simulink model "LKAS_DFL"  (R2018b)
settings: Solver=FixedStepDiscrete  StartTime=0.0  StopTime=10.0  FixedStep=0.01  RelTol=1e-3
InitFcn:
  | tmpVer = ver('MATLAB');
  | tmpVer = str2num(tmpVer.Version);
  | % -------------------------------------------------------------------
  | %  MATLAB file generated by Simulink.saveVars on 21-Nov-2019 10:06:14
  | %  MATLAB version: 7.13.0.564 (R2011b)
  | % -------------------------------------------------------------------
  | 
  | 
  | SInt16 = Simulink.AliasType;
  | SInt16.Description = 'Num';
  | if (tmpVer > 7.11)
  | 	SInt16.DataScope = 'Auto';
  | end
  | SInt16.HeaderFile = 'Rte_Type.h';
  | SInt16.BaseType = 'int16';
  | 
  | SInt32 = Simulink.AliasType;
  | SInt32.Description = 'Num';
  | if (tmpVer > 7.11)
  | 	SInt32.DataScope = 'Auto';
  | end
  | SInt32.HeaderFile = 'Rte_Type.h';
  | SInt32.BaseType = 'int32';
  | 
  | SInt8 = Simulink.AliasType;
  | SInt8.Description = 'Num';
  | if (tmpVer > 7.11)
  | 	SInt8.DataScope = 'Auto';
  | end
  | SInt8.HeaderFile = 'Rte_Type.h';
  | SInt8.BaseType = 'int8';
  | 
  | T_A_m2_1024_1_u32 = Simulink.NumericType;
  | T_A_m2_1024_1_u32.Description = 'm2 (square meters  (m2))';
  | if (tmpVer > 7.11)
  | 	T_A_m2_1024_1_u32.DataScope = 'Auto';
  | end
  | T_A_m2_1024_1_u32.HeaderFile = 'Rte_Type.h';
  | T_A_m2_1024_1_u32.DataTypeMode = 'Fixed-point: slope and bias scaling';
  | T_A_m2_1024_1_u32.SignednessBool = false;
  | T_A_m2_1024_1_u32.WordLength = 32;
  | T_A_m2_1024_1_u32.FixedExponent = -10;
  | T_A_m2_1024_1_u32.SlopeAdjustmentFactor = 1;
  | T_A_m2_1024_1_u32.Bias = 0;
  | T_A_m2_1024_1_u32.DataTypeOverride = 'Inherit';
  | T_A_m2_1024_1_u32.IsAlias = true;
  | 
  | T_A_m2_65536_1_u16 = Simulink.NumericType;
  | T_A_m2_65536_1_u16.Description = 'm2 (square meters  (m2))';
  | if (tmpVer > 7.11)
  | 	T_A_m2_65536_1_u16.DataScope = 'Auto';
  | end
  | T_A_m2_65536_1_u16.HeaderFile = 'Rte_Type.h';
  | T_A_m2_65536_1_u16.DataTypeMode = 'Fixed-point: slope and bias scaling';
  | T_A_m2_65536_1_u16.SignednessBool = false;
  | T_A_m2_65536_1_u16.WordLength = 16;
  | T_A_m2_65536_1_u16.FixedExponent = -16;
  | T_A_m2_65536_1_u16.SlopeAdjustmentFactor = 1;
  | T_A_m2_65536_1_u16.Bias = 0;
  | T_A_m2_65536_1_u16.DataTypeOverride = 'Inherit';
  | ... (+4598 lines)
StopFcn:
  | clear  T_A_m2_1024_1_u32 T_A_m2_65536_1_u16 T_A_m2_Float32 T_A_mm2_10_1_u16 T_A_mm2_4_1_s16 T_A_mm2_Float32 T_Cnt_Num_10_1_u32 T_Cnt_Num_1_1_s16 T_Cnt_Num_1_1_s32 T_Cnt_Num_1_1_s8 T_Cnt_Num_1_1_u16 T_Cnt_Num_1_1_u32 T_Cnt_Num_1_1_u8 T_E_J_1_1_s32 T_E_J_Float32 T_E_kJ_128_1_s32 T_E_kJ_Float32 T_E_kwh_10_1_u16 T_E_kwh_Float32 T_Epl_kwhpkm_100_1_u16 T_Epl_kwhpkm_Float32 T_F_N_1_1_s16 T_F_N_Float32 T_I_A_1000_1_u16 T_I_A_1048576_1_s32 T_I_A_2048_1_s16 T_I_A_32_1_s16 T_I_A_Float32 T_I_mA_1_1_s16 T_I_mA_32768_128_s16 T_I_mA_Float32 T_J_kgpm2_128_1_u16 T_J_kgpm2_Float32 T_K_NA_1000_1_s16 T_K_NA_100_1_s16 T_K_NA_100_1_u16 T_K_NA_1024_1_s16 T_K_NA_1024_1_u16 T_K_NA_128_1_s16 T_K_NA_128_1_u16 T_K_NA_128_1_u8 T_K_NA_16777216_1_u32 T_K_NA_16_1_s16 T_K_NA_16_1_u16 T_K_NA_16_1_u8 T_K_NA_1_16_u16 T_K_NA_1_1_s16 T_K_NA_1_1_u16 T_K_NA_1_1_u8 T_K_NA_32768_1_s16 T_K_NA_32768_1_u16 T_K_NA_32_1_s8 T_K_NA_4096_1_u16 T_K_NA_4194304_1_s32 T_K_NA_4194304_1_u16 T_K_NA_65536_1_s32 T_K_NA_65536_1_u16 T_K_NA_8192_1_s16 T_K_NA_8_1_s16 T_K_NA_Float32 T_M_Nm_16_1_s16 T_M_Nm_1_1_s16 T_M_Nm_32768_1_s16 T_M_Nm_32_1_s16 T_M_Nm_4_1_s16 T_M_Nm_512_1_s16 T_M_Nm_Float32 T_P_W_1_4_s16 T_P_W_1_8_s16 T_P_W_Float32 T_P_kW_128_1_s16 T_P_kW_1_8_s16 T_P_kW_8_1_s32 T_P_kW_Float32 T_Pct_pct_1024_1_s32 T_Pct_pct_1024_1_u32 T_Pct_pct_10_1_s16 T_Pct_pct_10_1_u32 T_Pct_pct_128_100_s8 T_Pct_pct_1_1_s16 T_Pct_pct_1_4_u8 T_Pct_pct_255_100_u16 T_Pct_pct_255_100_u8 T_Pct_pct_256_1_s16 T_Pct_pct_256_1_u16 T_Pct_pct_65535_100_u16 T_Pct_pct_Float32 T_R_ohm_1024_1_s16 T_R_ohm_32_1_s16 T_R_ohm_Float32 T_TK_K_16_1_s16 T_TK_K_Float32 T_T_degC_10_400_1_u16 T_T_degC_16_1_s16 T_T_degC_1_40_1_u8 T_T_degC_2_80_1_u8 T_T_degC_Float32 T_U_V_1000_1_u16 T_U_V_10_1_u8 T_U_V_200_1_u8 T_U_V_32_1_s16 T_U_V_4096_1_s16 T_U_V_512_1_s16 T_U_V_65535_8_u16 T_U_V_8192_1_u16 T_U_V_Float32 T_U_mV_1_1_s16 T_U_mV_256_20_u16 T_U_mV_Float32 T_V_l_256_1_s16 T_V_l_4096_1_s16 T_V_l_64_1_s16 T_V_l_65535_100_u16 T_V_l_Float32 T_V_ml_128_1_s16 T_V_ml_1_1_s16 T_V_ml_32768_1_s16 T_V_ml_Float32 T_V_ul_32_1_u16 T_V_ul_Float32 T_Vpl_clpkm_512_1_u16 T_Vpl_clpkm_Float32 T_a_kphps_16_1_s16 T_a_kphps_Float32 T_a_mps2_128_1_s16 T_a_mps2_Float32 T_c_MJpkg_256_1_s16 T_c_MJpkg_Float32 T_c_kJpgpK_1024_1_s16 T_c_kJpgpK_Float32 T_c_kJpkgpK_128_1_u16 T_c_kJpkgpK_Float32 T_chrg_Ah_1_1_s16 T_chrg_Ah_1_1_u16 T_chrg_Ah_1_1_u8 T_chrg_Ah_256_1_u16 T_chrg_Ah_4194304_1_s32 T_chrg_Ah_512_1_u16 T_chrg_Ah_8_1_u16 T_chrg_Ah_Float32 T_cmp_NA_100_1_s16 T_cmp_NA_128_1_s16 T_cmp_NA_16_1_s16 T_cmp_NA_32768_1_u16 T_cmp_NA_Float32 T_d2n_rpmps2_4_1_s16 T_d2n_rpmps2_Float32 T_dPct_pctps_16_1_s16 T_dPct_pctps_256_1_s16 T_dPct_pctps_Float32 T_dT_degCps_128_1_s16 T_dT_degCps_Float32 T_dV_lph_1_1_s16 T_dV_lph_Float32 T_dV_lpm_128_1_s16 T_dV_lpm_32_1_s16 T_dV_lpm_Float32 T_dV_lps_1024_1_u16 T_dV_lps_4_1_u16 T_dV_lps_Float32 T_dV_mlps_1024_1_s16 T_dV_mlps_Float32 T_d_BitField16 T_dm_gps_128_1_s16 T_dm_gps_128_1_u16 T_dm_gps_256_1_u16 T_dm_gps_Float32 T_dm_mgps_1_1_s16 T_dm_mgps_Float32 T_dn_rpmps_1_1_s16 T_dn_rpmps_2_1_s16 T_dn_rpmps_Float32 T_dp_Paps_1_1_s16 T_dp_Paps_Float32 T_dp_kPaps_1_1_s16 T_dp_kPaps_8_1_s16 T_dp_kPaps_Float32 T_dphi_degps_128_1_s16 T_dphi_degps_8_1_s16 T_dphi_degps_Float32 T_dr_ps_256_1_s16 T_dr_ps_Float32 T_drho_mgplps_1_2_s16 T_drho_mgplps_Float32 T_e_NA_1_1_u8 T_f_Hz_1_1_u16 T_f_Hz_1_1_u32 T_f_Hz_64_1_u16 T_f_Hz_8_1_s16 T_f_Hz_Float32 T_g_BitField32 T_l_km_16_1_s16 T_l_km_1_1_u16 T_l_km_1_1_u32 T_l_km_Float32 T_l_m_1024_1_s16 T_l_m_16_1_s16 T_l_m_1_1_u32 T_l_m_Float32 T_l_mm_16_1_s16 T_l_mm_1_1_u16 T_l_mm_4096_1_s16 T_l_mm_4_1_u8 T_l_mm_64_1_s16 T_l_mm_Float32 T_m_g_1_1_s16 T_m_g_2048_1_s16 T_m_g_32_1_u16 T_m_g_Float32 T_m_kg_1024_1_s16 T_m_kg_1_1_s16 T_m_kg_1_1_u32 T_m_kg_Float32 T_m_mg_128_1_s16 T_m_mg_32_1_s16 T_m_mg_Float32 T_n_rpm_1_1_s16 T_n_rpm_1_25_u8 T_n_rpm_256_50_u16 T_n_rpm_2_25_u8 T_n_rpm_4_1_u16 T_n_rpm_Float32 T_p_MPa_64_1_s16 T_p_MPa_Float32 T_p_Pa_1_1_s16 T_p_Pa_Float32 T_p_kPa_1_10_u16 T_p_kPa_1_1_s16 T_p_kPa_1_1_u8 T_p_kPa_256_1_u16 T_p_kPa_32_1_u16 T_p_kPa_64_1_s16 T_p_kPa_Float32 T_phi_deg_100_1_s16 T_phi_deg_1024_1_s16 T_phi_deg_128_1_s16 T_phi_deg_1_1_u8 T_phi_deg_256_1_s16 T_phi_deg_2_1_s8 T_phi_deg_32_1_s16 T_phi_deg_512_6_s32 T_phi_deg_Float32 T_phi_rad_2048_1_s16 T_phi_rad_Float32 T_r_NA_1024_1_s16 T_r_NA_1024_1_u16 T_r_NA_16384_1_s16 T_r_NA_16_1_s16 T_r_NA_256_1_s8 T_r_NA_256_1_u16 T_r_NA_32768_1_u16 T_r_NA_32_1_u16 T_r_NA_4096_1_s16 T_r_NA_65535_2_u16 T_r_NA_8192_1_u16 T_r_NA_Float32 T_rho_gpl_8192_1_s16 T_rho_gpl_Float32 T_rho_kgpm3_16_1_s16 T_rho_kgpm3_Float32 T_rho_mgpl_1_1_s16 T_rho_mgpl_64_1_s16 T_rho_mgpl_Float32 T_t_hour_1_1_s16 T_t_hour_Float32 T_t_m_1_1_u16 T_t_m_Float32 T_t_ms_1_1_s16 T_t_ms_1_1_u16 T_t_ms_1_1_u32 T_t_ms_4096_1_s16 T_t_ms_64_1_s16 T_t_ms_Float32 T_t_s_1000_1_s16 T_t_s_100_1_s16 T_t_s_10_1_s16 T_t_s_10_1_u16 T_t_s_1_1_s16 T_t_s_1_1_u16 T_t_s_1_1_u32 T_t_s_Float32 T_t_us_10_1_u32 T_t_us_1_1_s16 T_t_us_1_1_u32 T_t_us_1_4_u16 T_t_us_Float32 T_v_kph_1_1_u8 T_v_kph_64_1_s16 T_v_kph_64_1_u16 T_v_kph_Float32 T_v_mps_256_1_s16 T_v_mps_Float32 T_w_radps_32_1_s16 T_w_radps_Float32 T_y_BitField8 T_y_BitFieldDiagProgress T_y_BitFieldDiagStatus T_y_NA_1_1_u8 SInt16 SInt32 SInt8 T_BOOLEAN UInt16 UInt32 UInt8 s16 s32 s8 u16 u32 u8
model workspace (MAT data in the model file):
  MCOS : class17 (value not decoded)
  MCOS : class17 (value not decoded)
  MCOS : class17 (value not decoded)
  MCOS : class17 (value not decoded)
  MCOS : class17 (value not decoded)
  MCOS : class17 (value not decoded)
  MCOS : class17 (value not decoded)
  MCOS : class17 (value not decoded)
  MCOS : class17 (value not decoded)
  MCOS : class17 (value not decoded)
  MCOS : class17 (value not decoded)
  MCOS : class17 (value not decoded)
  MCOS : class17 (value not decoded)
  MCOS : class17 (value not decoded)
  MCOS : class17 (value not decoded)
  MCOS : class17 (value not decoded)
  MCOS : class17 (value not decoded)
  MCOS : class17 (value not decoded)
  MCOS : class17 (value not decoded)
  MCOS : class17 (value not decoded)
  MCOS : class17 (value not decoded)
  MCOS : class17 (value not decoded)
  MCOS : class17 (value not decoded)
  MCOS : class17 (value not decoded)
  MCOS : class17 (value not decoded)
  MCOS : class17 (value not decoded)
  MCOS : class17 (value not decoded)
  MCOS : class17 (value not decoded)
  MCOS : class17 (value not decoded)
  MCOS : class17 (value not decoded)
  MCOS : class17 (value not decoded)
  MCOS : class17 (value not decoded)
  MCOS : class17 (value not decoded)
  MCOS : class17 (value not decoded)
  MCOS : class17 (value not decoded)
  MCOS : class17 (value not decoded)
  MCOS : class17 (value not decoded)
  MCOS : class17 (value not decoded)
  MCOS : class17 (value not decoded)
  MCOS : class17 (value not decoded)
  MCOS : class17 (value not decoded)
  MCOS : class17 (value not decoded)
  MCOS : class17 (value not decoded)
  MCOS : class17 (value not decoded)
  MCOS : class17 (value not decoded)
  MCOS : class17 (value not decoded)
  MCOS : class17 (value not decoded)
  MCOS : class17 (value not decoded)
  MCOS : class17 (value not decoded)
  MCOS : class17 (value not decoded)
  MCOS : class17 (value not decoded)
  MCOS : class17 (value not decoded)
  MCOS : class17 (value not decoded)
  MCOS : class17 (value not decoded)
  MCOS : class17 (value not decoded)
  MCOS : class17 (value not decoded)
  MCOS : class17 (value not decoded)
  MCOS : class17 (value not decoded)
  MCOS : class17 (value not decoded)
  MCOS : class17 (value not decoded)
  MCOS : class17 (value not decoded)
  MCOS : class17 (value not decoded)
  MCOS : class17 (value not decoded)
  MCOS : class17 (value not decoded)
  MCOS : class17 (value not decoded)
  MCOS : class17 (value not decoded)
  MCOS : class17 (value not decoded)
  MCOS : class17 (value not decoded)
  MCOS : class17 (value not decoded)
  MCOS : class17 (value not decoded)
  MCOS : class17 (value not decoded)
  MCOS : class17 (value not decoded)
  MCOS : class17 (value not decoded)
  MCOS : class17 (value not decoded)
  MCOS : class17 (value not decoded)
  MCOS : class17 (value not decoded)
  MCOS : class17 (value not decoded)
  MCOS : class17 (value not decoded)
  MCOS : class17 (value not decoded)
  MCOS : class17 (value not decoded)
  MCOS : class17 (value not decoded)
  MCOS : class17 (value not decoded)
  MCOS : class17 (value not decoded)
  MCOS : class17 (value not decoded)
  MCOS : class17 (value not decoded)
  MCOS : class17 (value not decoded)
  MCOS : class17 (value not decoded)
  MCOS : class17 (value not decoded)
  MCOS : class17 (value not decoded)
  MCOS : class17 (value not decoded)
  MCOS : class17 (value not decoded)
  MCOS : class17 (value not decoded)
  MCOS : class17 (value not decoded)
  MCOS : class17 (value not decoded)
  MCOS : class17 (value not decoded)
  MCOS : class17 (value not decoded)
  MCOS : class17 (value not decoded)
  MCOS : class17 (value not decoded)
  MCOS : class17 (value not decoded)
  MCOS : class17 (value not decoded)
  MCOS : class17 (value not decoded)
  MCOS : class17 (value not decoded)
  MCOS : class17 (value not decoded)
  MCOS : class17 (value not decoded)
  MCOS : class17 (value not decoded)
  MCOS : class17 (value not decoded)
undefined symbols (not defined in the file): LKA_CarWidth, LKA_SampleTime, LKA_StrRatio_C, LKA_Veh2CamL_C, LKA_Veh2CamW_C, LKA_WhlBaseL_C, LL_CompSWA_C, LL_CrvtPrvwT_C, LL_DesDvt_C, LL_DvtComp_C, LL_DvtPrvwT_C, LL_DvtSpdDet_vDvtSpdMin_C, LL_HdAgExT_C, LL_HdAgPrvwT_C, LL_LAccMax_C, LL_LAccRMax_C, LL_Laneline_Select, LL_LDW_EarliestWarnLine_C, LL_LDW_LatestWarnLine_C, LL_LDWS_SUPPRESS_HEADING, LL_LFClb_TFC_DiffCtlBalance, LL_LFClb_TFC_DiffCtrlMaxSWA, LL_LFClb_TFC_DiffCtrlRatio, LL_LFClb_TFC_facmGainLutGain1_C, LL_LFClb_TFC_facmGainLutGain2_C, LL_LFClb_TFC_facmIntegRatio, LL_LFClb_TFC_facmKlat_C, LL_LFClb_TFC_FfCtlRatio_C, LL_LFClb_TFC_phiIntegCtlMaxSWA_C, LL_LFClb_TFC_tiKlatPrvwT_C, LL_LFClb_TFC_vGainLutVehSpdLwr_C, LL_LFClb_TFC_vGainLutVehSpdUpr_C, LL_LKA_EarliestWarnLine_C, LL_LKA_LatestWarnLine_C, LL_LKA_SWATrq_Kf_Switch, LL_LKA_SWATrq_KfA, LL_LKA_SWATrq_KfB, LL_LKA_SWATrq_KiA, LL_LKA_SWATrq_KiB, LL_LKA_SWATrq_KiMax, LL_LKA_SWATrq_Kp, LL_LKAExPrcs_ExitC0Dvt, LL_LKAExPrcs_ExitC0Swt, LL_LKAExPrcs_tiExitTime1, LL_LKAExPrcs_tiExitTime2, LL_LKAExPrcs_tiExitTime3, LL_LKAS_OUT_OF_CONTROL_LAT_VEL, LL_LKAS_OUT_OF_CONTROL_TTLC, LL_LKASWASyn_M0, LL_LKASWASyn_M1, LL_LKASWASyn_M2, LL_LKASWASyn_M3K, LL_LKASWASyn_SWAaddMax, LL_LKASWASyn_T2, LL_LKASWASyn_tiTrqSwaRtTime, LL_LKASWASyn_tiTrqSwaTime, LL_LKASWASyn_TrqMax, LL_LKASWASyn_TrqSwaAddSwt, LL_LKASWASyn_TrqSwaRateDiff, LL_LSpdCompT_C ... (+42)
libraries: simulink x137, dspstat3 x3, simulink_extras x1
(part 9 of 19)

== system LKAS_DFL/LKAS/LL/LLOn/LKA/Driver Torque Addition (DTA)/Subsystem ==
  DTA_bsInInfoSyn : Inport
  DTA_bsLFClb : Inport  Port=2
  Enable : EnablePort
      settings: AttributesFormatString=states = %<StatesWhenEnabling>
  Add : Sum
  Bus Selector2 : BusSelector  OutputSignals=bsVehMovInfo.ESC_VehSpd,bsEPSInfo.EPS_SW_Trq,bsLaneInfo.bsL0Info.L0_C0,bsLaneInfo.bsR0Info.R0_C0
  Bus Selector4 : BusSelector  OutputSignals=bsLKAClb.LL_LKASWAClb.LL_LKASWASyn_SWAaddMax,bsLKAClb.LL_LKASWAClb.LL_LKASWASyn_TrqMax,bsLKAClb.LL_LKASWAClb.LL_LKASWASyn_TrqSwaAddSwt,bsLKAClb.LL_LKASWAClb.LL_LKASWASyn_tiTrqSwaTime,bsLKAClb.LL_LKASWAClb.LL_LKASWASyn_tiTrqSwaRtTime,bsLKAClb.LL_LKASWAClb.LL_LKASWASyn_TrqSwaRateDiff,bsConstantClb.LKA_SampleTime
  Constant1 : Constant  Value=5  OutDataTypeStr=single
  Constant2 : Constant  Value=-5  OutDataTypeStr=single
  Divide1 : Product  Inputs=***
  Divide3 : Product  Inputs=**
  DriverSwaTrqAdd : MATLAB Function  TreatAsAtomicUnit=on
  LowPass : Subsystem
  LowPass1 : Subsystem
  Rate Limiter Dynamic : simulink/Discontinuities/Rate Limiter Dynamic
      settings: SourceProductName=Simulink
  Saturation : Saturate  UpperLimit=30  LowerLimit=-30
      settings: AttributesFormatString="Min = %<LowerLimit>  Max = %<UpperLimit>"
  Out1 : Outport  OutputWhenDisabled=reset  InitialOutput=0
      settings: AttributesFormatString=%<OutputWhenDisabled> = %<InitialOutput>
  wires:
  Add/1 -> Rate Limiter Dynamic/2
  Bus Selector4/3 -> Divide3/1, Divide1/1  "<LL_LKASWASyn_TrqSwaAddSwt>"
  LowPass1/1(y) -> Saturation/1  "SWARateAdd"
  Divide3/1 -> Add/1  "TrqSWAAdd"
  Constant2/1 -> Rate Limiter Dynamic/3
  Bus Selector4/1 -> DriverSwaTrqAdd/5(swaaddmax)  "<LL_LKASWASyn_SWAaddMax>"
  Constant1/1 -> Rate Limiter Dynamic/1
  DriverSwaTrqAdd/1(Swaadd) -> LowPass/2(u)  "TrqSWAAddRaw"
  Rate Limiter Dynamic/1 -> Out1/1
  Saturation/1 -> Divide1/2
  DTA_bsInInfoSyn/1 -> Bus Selector2/1
  Bus Selector4/4 -> LowPass/1(T)  "<LL_LKASWASyn_tiTrqSwaTime>"
  LowPass/1(y) -> Divide3/2, LowPass1/2(u)  "TrqSWAAdd"
  Divide1/1 -> Add/2  "SWARateAdd"
  Bus Selector2/2 -> DriverSwaTrqAdd/2(trq)  "<EPS_SW_Trq>"
  Bus Selector2/4 -> DriverSwaTrqAdd/4(r0c0)  "<R0_C0>"
  Bus Selector4/6 -> Divide1/3  "<LL_LKASWASyn_TrqSwaRateDiff>"
  Bus Selector2/1 -> DriverSwaTrqAdd/1(spd)  "<ESC_VehSpd>"
  Bus Selector4/5 -> LowPass1/1(T)  "<LL_LKASWASyn_tiTrqSwaRtTime>"
  Bus Selector2/3 -> DriverSwaTrqAdd/3(l0c0)  "<L0_C0>"
  Bus Selector4/7 -> LowPass1/3(dT), LowPass/3(dT)  "<LKA_SampleTime>"
  Bus Selector4/2 -> DriverSwaTrqAdd/6(trqmax)  "<LL_LKASWASyn_TrqMax>"
  DTA_bsLFClb/1 -> Bus Selector4/1

== system LKAS_DFL/LKAS/LL/LLOn/LKA/Driver Torque Addition (DTA)/Subsystem1 ==
  DTA_bsInInfoSyn : Inport
  DTA_bsLFClb : Inport  Port=2
  Add1 : Sum  Inputs=-+
  Bus Selector : BusSelector  OutputSignals=bsEPSInfo.EPS_SW_Trq
  Bus Selector1 : BusSelector  OutputSignals=bsLKAClb.LL_LKASWAClb.LL_LKASWASyn_M3K,bsLKAClb.LL_LKASWAClb.LL_LKASWASyn_M0,bsLKAClb.LL_LKASWAClb.LL_LKASWASyn_M1,bsLKAClb.LL_LKASWAClb.LL_LKASWASyn_M2,bsLKAClb.LL_LKASWAClb.LL_LKASWASyn_T2
  Divide : Product  Inputs=**
  MATLAB Function : MATLAB Function  TreatAsAtomicUnit=on
  Moving Standard Deviation2 : Subsystem  TreatAsAtomicUnit=on
      mask Display: disp(['Moving' char(10) 'Standard' char(10) 'Deviation']);
  Saturation1 : Saturate  UpperLimit=0.2  LowerLimit=0
      settings: AttributesFormatString="Min = %<LowerLimit>  Max = %<UpperLimit>"
  Saturation2 : Saturate  UpperLimit=1  LowerLimit=0
      settings: AttributesFormatString="Min = %<LowerLimit>  Max = %<UpperLimit>"
  TickTime (TTime) : Subsystem
      mask Display:
      | port_label('output', 1, 'TTime');
      | color('blue');
      | text(0.98,0.9,'VCDC Block','horizontalAlignment','right');
      | color('black');
      | text(0.5,0.55,'Tick Time','horizontalAlignment','center');
      | text(0.5,0.4,'(TTime)','horizontalAlignment','center');
  Out1 : Outport
  wires:
  Bus Selector1/2 -> MATLAB Function/1(M0)  "<LL_LKASWASyn_M0>"
  Bus Selector1/3 -> MATLAB Function/2(M1)  "<LL_LKASWASyn_M1>"
  [PT1] -> MATLAB Function/4(T1)
  [T] -> MATLAB Function/6(T)
  Saturation1/1 -> Add1/1  "M3"
  MATLAB Function/1(M) -> Add1/2
  Bus Selector1/5 -> MATLAB Function/5(T2)  "<LL_LKASWASyn_T2>"
  TickTime (TTime)/1(Out1) -> [T]
  Divide/1 -> Saturation1/1
  Add1/1 -> Saturation2/1
  Bus Selector1/1 -> Divide/2  "<LL_LKASWASyn_M3K>"
  Bus Selector1/4 -> MATLAB Function/3(M2)  "<LL_LKASWASyn_M2>"
  Bus Selector/1 -> Moving Standard Deviation2/1(In1)  "<EPS_SW_Trq>"
  Moving Standard Deviation2/1(Out1) -> Divide/1
  DTA_bsInInfoSyn/1 -> Bus Selector/1
  DTA_bsLFClb/1 -> Bus Selector1/1
  Saturation2/1 -> Out1/1

== system LKAS_DFL/LKAS/LL/LLOn/LKA/LKA Exit Processing (LKAExPrcs)/Exit Time 1 ==
  bsLKAInPInfo : Inport
  bsLKAClb : Inport  Port=2
  Abs : Abs
  Add : Sum
  Add2 : Sum  OutDataTypeStr=single
  Bus Selector1 : BusSelector  OutputSignals=bsConstantClb.LKA_SampleTime,bsLKAClb.LL_LKAExPrcs.LL_LKAExPrcs_tiExitTime1
  Bus Selector2 : BusSelector  OutputSignals=bsPrCrvtInfo.crPrvwCrvt
  Constant : Constant  Value=0.004  OutDataTypeStr=single
  Constant1 : Constant  Value=0.5  OutDataTypeStr=single
  Divide : Product  Inputs=***/
  Memory : Memory  InheritSampleTime=on
  Relational Operator4 : RelationalOperator  OutDataTypeStr=boolean  RndMeth=Nearest
  Saturation : Saturate  UpperLimit=0.004  LowerLimit=0
      settings: AttributesFormatString="Min = %<LowerLimit>  Max = %<UpperLimit>"
  Saturation2 : Saturate  UpperLimit=20  LowerLimit=0
      settings: AttributesFormatString="Min = %<LowerLimit>  Max = %<UpperLimit>"
  Exit1 : Outport
  wires:
  Saturation2/1 -> Relational Operator4/1, Memory/1
  Bus Selector1/1 -> Add2/1  "<LKA_SampleTime>"
  bsLKAClb/1 -> Bus Selector1/1
  Add2/1 -> Saturation2/1
  Memory/1 -> Add2/2
  Relational Operator4/1 -> Exit1/1
  bsLKAInPInfo/1 -> Bus Selector2/1
  Constant/1 -> Divide/4
  Constant1/1 -> Divide/2
  Bus Selector2/1 -> Abs/1  "<crPrvwCrvt>"
  Divide/1 -> Add/2
  Abs/1 -> Saturation/1
  Add/1 -> Relational Operator4/2
  Saturation/1 -> Divide/3
  Bus Selector1/2 -> Add/1, Divide/1  "<LL_LKAExPrcs_tiExitTime1>"

== system LKAS_DFL/LKAS/LL/LLOn/LKA/LKA Exit Processing (LKAExPrcs)/Exit Time 2 ==
  bsLKAClb : Inport
  bsLKAInPInfo : Inport  Port=2
  T1 : Inport  Port=3
  Abs : Abs
  Abs2 : Abs
  Abs3 : Abs
  Add1 : Sum
  Add2 : Sum  OutDataTypeStr=single
  Add3 : Sum  Inputs=+-
  Bus Selector1 : BusSelector  OutputSignals=bsPrCrvtInfo.crPrvwCrvt
  Bus Selector3 : BusSelector  OutputSignals=bsConstantClb.LKA_SampleTime,bsConstantClb.LKA_CarWidth,bsLKAClb.LL_LKAExPrcs.LL_LKAExPrcs_tiExitTime2
  Bus Selector4 : BusSelector  OutputSignals=bsDvtInfo.ILftDvt,bsDvtInfo.IRgtDvt,LaneWidth
  Constant : Constant  Value=0.004  OutDataTypeStr=single
  Constant1 : Constant  Value=0.5  OutDataTypeStr=single
  Divide : Product  Inputs=***/
  Gain : Gain  Gain=1/6
  Logical Operator1 : Logic  Inputs=3  AllPortsSameDT=off  OutDataTypeStr=boolean
  Memory : Memory  InheritSampleTime=on
  Relational Operator2 : RelationalOperator  OutDataTypeStr=boolean  RndMeth=Nearest
  Relational Operator3 : RelationalOperator  OutDataTypeStr=boolean  RndMeth=Nearest
  Relational Operator4 : RelationalOperator  OutDataTypeStr=boolean  RndMeth=Nearest
  Saturation : Saturate  UpperLimit=0.004  LowerLimit=0
      settings: AttributesFormatString="Min = %<LowerLimit>  Max = %<UpperLimit>"
  Saturation2 : Saturate  UpperLimit=12  LowerLimit=0
      settings: AttributesFormatString="Min = %<LowerLimit>  Max = %<UpperLimit>"
  Sum Condition1 : Subsystem
  Exit2 : Outport
  wires:
  Add3/1 -> Gain/1
  Bus Selector4/3 -> Add3/1  "<LaneWidth>"
  Bus Selector4/2 -> Abs3/1  "<IRgtDvt>"
  Bus Selector4/1 -> Abs2/1  "<ILftDvt>"
  Saturation2/1 -> Relational Operator4/1, Memory/1
  Gain/1 -> Relational Operator2/2, Relational Operator3/2
  Abs3/1 -> Relational Operator3/1
  Relational Operator2/1 -> Logical Operator1/2
  Abs2/1 -> Relational Operator2/1
  Relational Operator3/1 -> Logical Operator1/3
  Logical Operator1/1 -> Sum Condition1/Enable
  Add2/1 -> Saturation2/1
  Relational Operator4/1 -> Logical Operator1/1
  Memory/1 -> Add2/2
  Bus Selector3/1 -> Sum Condition1/1(Sample Time), Add2/1  "<LKA_SampleTime>"
  T1/1 -> Relational Operator4/2
  Sum Condition1/1(Out) -> Exit2/1
  bsLKAInPInfo/1 -> Bus Selector1/1, Bus Selector4/1
  Bus Selector1/1 -> Abs/1  "<crPrvwCrvt>"
  Add1/1 -> Sum Condition1/2(Time Exit 2)
  Constant/1 -> Divide/4
  Abs/1 -> Saturation/1
  Constant1/1 -> Divide/2
  Divide/1 -> Add1/2
  Saturation/1 -> Divide/3
  bsLKAClb/1 -> Bus Selector3/1
  Bus Selector3/2 -> Add3/2  "<LKA_CarWidth>"
  Bus Selector3/3 -> Add1/1, Divide/1  "<LL_LKAExPrcs_tiExitTime2>"

== system LKAS_DFL/LKAS/LL/LLOn/LKA/LKA Exit Processing (LKAExPrcs)/Exit Time 3 ==
  bsLKAInPInfo : Inport
  bsLKAClb : Inport  Port=2
  T1 : Inport  Port=3
  Abs4 : Abs
  Add : Sum  Inputs=+-
  Add2 : Sum  OutDataTypeStr=single
  Add6 : Sum
  Bus Selector3 : BusSelector  OutputSignals=bsConstantClb.LKA_SampleTime,bsConstantClb.LKA_CarWidth,bsLKAClb.LL_LKAExPrcs.LL_LKAExPrcs_tiExitTime3,bsLKAClb.LL_LKAExPrcs.LL_LKAExPrcs_ExitC0Dvt,bsLKAClb.LL_LKAExPrcs.LL_LKAExPrcs_ExitC0Swt
  Bus Selector4 : BusSelector  OutputSignals=bsPrCrvtInfo.crPrvwCrvt
  Bus Selector5 : BusSelector  OutputSignals=LaneWidth,bsDvtInfo.ILftDvt,bsDvtInfo.IRgtDvt
  Constant : Constant  Value=0.004  OutDataTypeStr=single
  Constant7 : Constant  Value=2  OutDataTypeStr=single
  Divide1 : Product  Inputs=**/
  Gain : Gain  Gain=1/3
  Logical Operator1 : Logic  Inputs=3  AllPortsSameDT=off  OutDataTypeStr=boolean
  Logical Operator2 : Logic  Inputs=4  AllPortsSameDT=off  OutDataTypeStr=boolean
  Memory : Memory  InheritSampleTime=on
  Moving Standard Deviation1 : Subsystem  TreatAsAtomicUnit=on
      mask Display: disp(['Moving' char(10) 'Standard' char(10) 'Deviation']);
  Moving Standard Deviation2 : Subsystem  TreatAsAtomicUnit=on
      mask Display: disp(['Moving' char(10) 'Standard' char(10) 'Deviation']);
  Relational Operator2 : RelationalOperator  OutDataTypeStr=boolean  RndMeth=Nearest
  Relational Operator3 : RelationalOperator  OutDataTypeStr=boolean  RndMeth=Nearest
  Relational Operator4 : RelationalOperator  OutDataTypeStr=boolean  RndMeth=Nearest
  Relational Operator5 : RelationalOperator  Operator=<=  OutDataTypeStr=boolean  RndMeth=Nearest
  Relational Operator6 : RelationalOperator  Operator=<=  OutDataTypeStr=boolean  RndMeth=Nearest
  Saturation : Saturate  UpperLimit=0.004  LowerLimit=0
      settings: AttributesFormatString="Min = %<LowerLimit>  Max = %<UpperLimit>"
  Saturation2 : Saturate  UpperLimit=10  LowerLimit=0
      settings: AttributesFormatString="Min = %<LowerLimit>  Max = %<UpperLimit>"
  Sum Condition : Subsystem
  Sum Condition1 : Subsystem
  Exit3 : Outport
  wires:
  Gain/1 -> Relational Operator2/2, Relational Operator3/2
  Bus Selector5/1 -> Add/1  "<LaneWidth>"
  Bus Selector5/2 -> Moving Standard Deviation2/1(In1), Relational Operator2/1  "<ILftDvt>"
  Bus Selector5/3 -> Relational Operator3/1, Moving Standard Deviation1/1(In1)  "<IRgtDvt>"
  T1/1 -> Relational Operator4/2
  [LKA_SampleTime] -> Add2/1
  Memory/1 -> Add2/2
  Add2/1 -> Saturation2/1
  Relational Operator4/1 -> Logical Operator1/1
  Saturation2/1 -> Relational Operator4/1, Memory/1
  Logical Operator1/1 -> Logical Operator2/1
  Relational Operator3/1 -> Logical Operator1/3
  Relational Operator2/1 -> Logical Operator1/2
  Add/1 -> Gain/1
  bsLKAClb/1 -> Bus Selector3/1
  Logical Operator2/1 -> Exit3/1
  Moving Standard Deviation2/1(Out1) -> Relational Operator5/1
  Relational Operator5/1 -> Sum Condition/Enable
  Sum Condition/1(Out) -> Logical Operator2/3
  Sum Condition1/1(Out) -> Logical Operator2/2
  Relational Operator6/1 -> Sum Condition1/Enable
  Add6/1 -> Sum Condition/2(In1), Sum Condition1/2(In1)
  Moving Standard Deviation1/1(Out1) -> Relational Operator6/1
  bsLKAInPInfo/1 -> Bus Selector4/1, Bus Selector5/1
  Constant/1 -> Divide1/3
  Divide1/1 -> Add6/2
  Abs4/1 -> Saturation/1
  Saturation/1 -> Divide1/2
  Bus Selector4/1 -> Abs4/1  "<crPrvwCrvt>"
  Constant7/1 -> Divide1/1
  [LKA_SampleTime] -> Sum Condition1/1(In), Sum Condition/1(In)
  Bus Selector3/5 -> Logical Operator2/4  "<LL_LKAExPrcs_ExitC0Swt>"
  Bus Selector3/4 -> Relational Operator6/2, Relational Operator5/2  "<LL_LKAExPrcs_ExitC0Dvt>"
  Bus Selector3/3 -> Add6/1  "<LL_LKAExPrcs_tiExitTime3>"
  Bus Selector3/2 -> Add/2  "<LKA_CarWidth>"
  Bus Selector3/1 -> [LKA_SampleTime]  "<LKA_SampleTime>"

== system LKAS_DFL/LKAS/LL/LLOn/LKA/LKA Motion Planning (LKAMP) /LKA Motion Planning Calculation (LKAMPCal) ==
  LKAMPCal_bsLKAInPInfo : Inport
  LKAMPCal_bsLKAClb : Inport  Port=2
  Action Port : ActionPort  InitializeStates=reset
      settings: AttributesFormatString=states = %<InitializeStates>
  Bus Creator : BusCreator  Inputs=6
  Bus Creator3 : BusCreator  Inputs=5
  Bus Selector : BusSelector  OutputSignals=MPInP_stLDDir,MPInP_tiTTLCIni,MPInP_vVehSpdIni,MPInP_phiSWAIni,MPInP_phiPrvwHdAgIni,MPInP_phiHdAgIni,MPInP_phiHdAgMax,MPInP_lDvtIni,UndrLim_dphiSWARMax,StbFacm_SY
  Bus Selector1 : BusSelector  OutputSignals=bsConstantClb.LKA_WhlBaseL_C,bsConstantClb.LKA_StrRatio_C,bsLKAClb.LL_DesDvt_C,bsLKAClb.LL_lStpLngth_C
  Bus Selector3 : BusSelector  OutputSignals=signal1,signal2,signal3,signal4,signal5
  MATLAB Function : MATLAB Function  TreatAsAtomicUnit=on
  Memory{,1..4} (5 alike) : Memory  InheritSampleTime=on
  Time Division (TDiv) : Subsystem
  Time Division (TDiv)1 : Subsystem
  Time Division (TDiv)2 : Subsystem
  Time Division (TDiv)3 : Subsystem
  Time Division (TDiv)4 : Subsystem
  LKAMPCal_bsLKAMPCalOut : Outport
      settings: AttributesFormatString=%<OutputWhenDisabled> = %<InitialOutput>
  wires:
  Time Division (TDiv)4/1(Out2) -> Bus Creator3/5
  Time Division (TDiv)3/1(Out2) -> Bus Creator3/4
  Time Division (TDiv)2/1(Out2) -> Bus Creator3/3
  Time Division (TDiv)1/1(Out2) -> Bus Creator3/2
  Time Division (TDiv)/1(Out1) -> Bus Creator3/1
  Memory4/1 -> Time Division (TDiv)4/1(TDiv_bsTDivInfoOut1)
  MATLAB Function/11(K1K2Det_bsTDivInfoOut_Ph2SWAIni) -> Memory4/1
  MATLAB Function/10(K1K2Det_bsTDivInfoOut_Ph2DvtEnd) -> Memory3/1
  Memory3/1 -> Time Division (TDiv)3/1(TDiv_bsTDivInfoOut1)
  Memory2/1 -> Time Division (TDiv)2/1(TDiv_bsTDivInfoOut1)
  MATLAB Function/9(K1K2Det_bsTDivInfoOut_Mode2Num) -> Memory2/1
  MATLAB Function/8(K1K2Det_bsTDivInfoOut_Mode1Num) -> Memory1/1
  Memory1/1 -> Time Division (TDiv)1/1(TDiv_bsTDivInfoOut1)
  Bus Creator3/1 -> Bus Selector3/1
  Memory/1 -> Time Division (TDiv)/1(TDiv_bsTDivInfoOut)
  MATLAB Function/7(K1K2Det_bsTDivInfoOut_ModeFlg) -> Memory/1
  Bus Selector3/5 -> MATLAB Function/16(K1K2Det_bsTDivInfo_Ph2SWAIni)  "<signal5>"
  Bus Selector3/2 -> MATLAB Function/13(K1K2Det_bsTDivInfo_Mode1Num)  "<signal2>"
  Bus Selector3/1 -> MATLAB Function/12(K1K2Det_bsTDivInfo_ModeFlg)  "<signal1>"
  Bus Selector3/3 -> MATLAB Function/14(K1K2Det_bsTDivInfo_Mode2Num)  "<signal3>"
  Bus Selector3/4 -> MATLAB Function/15(K1K2Det_bsTDivInfo_Ph2DvtEnd)  "<signal4>"
  Bus Selector/9 -> MATLAB Function/10(K1K2Det_dphiSWARMax)  "<UndrLim_dphiSWARMax>"
  MATLAB Function/6(K1K2Det_dphi1PhHdAgIni) -> Bus Creator/6
  Bus Selector/5 -> MATLAB Function/5(K1K2Det_phiPrvwHdAgIni)  "<MPInP_phiPrvwHdAgIni>"
  Bus Selector/6 -> MATLAB Function/7(K1K2Det_phi1PhDesHdAgIni)  "<MPInP_phiHdAgIni>"
  Bus Selector/2 -> MATLAB Function/2(K1K2Det_tiTTLC0)  "<MPInP_tiTTLCIni>"
  MATLAB Function/4(K1K2Det_phi2PhSWAIni) -> Bus Creator/4  "K1K2Det_phi2PhSWAIni"
  Bus Selector/4 -> MATLAB Function/4(K1K2Det_phiIniSWA)  "<MPInP_phiSWAIni>"
  Bus Selector/8 -> MATLAB Function/9(K1K2Det_l1PhDvtIni)  "<MPInP_lDvtIni>"
  Bus Selector/10 -> MATLAB Function/21(K1K2Det_bsSysCfg_SY_StbFacm_SY)  "<StbFacm_SY>"
  Bus Selector/1 -> MATLAB Function/1(K1K2Det_stLDDir)  "<MPInP_stLDDir>"
  Bus Selector/7 -> MATLAB Function/8(K1K2Det_phi2PhDesHdAg)  "<MPInP_phiHdAgMax>"
  Bus Selector/3 -> MATLAB Function/3(K1K2Det_vVehSpd)  "<MPInP_vVehSpdIni>"
  MATLAB Function/1(K1K2Det_dphi1PhSWAGrad) -> Bus Creator/1
  MATLAB Function/3(K1K2Det_dphi2PhSWAGrad2) -> Bus Creator/3
  MATLAB Function/5(K1K2Det_stReplFlag) -> Bus Creator/5
  MATLAB Function/2(K1K2Det_dphi2PhSWAGrad1) -> Bus Creator/2
  Bus Creator/1 -> LKAMPCal_bsLKAMPCalOut/1  "LKAMPCal_bsLKAMPCalOut"
  LKAMPCal_bsLKAClb/1 -> Bus Selector1/1
  LKAMPCal_bsLKAInPInfo/1 -> Bus Selector/1
  Bus Selector1/1 -> MATLAB Function/19(K1K2Det_bsSysCfg_SY_WhlBase_SY)  "<LKA_WhlBaseL_C>"
  Bus Selector1/2 -> MATLAB Function/20(K1K2Det_bsSysCfg_SY_StRatio_SY)  "<LKA_StrRatio_C>"
  Bus Selector1/3 -> MATLAB Function/17(K1K2Det_lDesDvt)  "<LL_DesDvt_C>"
  Bus Selector1/4 -> MATLAB Function/18(K1K2Det_lStpLngth)  "<LL_lStpLngth_C>"

== system LKAS_DFL/LKAS/LL/LLOn/LKA/LKA Motion Planning (LKAMP) /Motion Planning Input Processing (MPInP) ==
  MPInP_stLKAActvFlg : Inport
  MPInP_phiHdAgMax : Inport  Port=2
  MPInP_bsLKAInPInfo : Inport  Port=3
  MPInP_bsInInfoSyn : Inport  Port=4
  Bus Creator : BusCreator  Inputs=11
  Bus Selector1 : BusSelector  OutputSignals=bsTTLCInfo.LFTTTLC,bsTTLCInfo.RGTTTLC
  Bus Selector3 : BusSelector  OutputSignals=bsSWAInfo.SW_Angle,bsVehMovInfo.ESC_VehSpd
  Bus Selector4 : BusSelector  OutputSignals=bsPrHdAgInfo.phiPrvwTTLCHdAgLft,bsPrHdAgInfo.phiPrvwTTLCHdAgRgt,bsPrDvtInfo.lPrvwDvtLft,bsPrDvtInfo.lPrvwDvtRgt,bsHdAgInfo.phiHdAg,bsUndrLimInfo.UndrLim_dphiSWARMax
  Cast To Single1 : DataTypeConversion  LockScale=on
  Constant : Constant  Value=0.09  OutDataTypeStr=single
  Divide1 : Product  Inputs=*/
  Lane Information Selection (LaneInfoSel) : Subsystem
  Lane Information Selection (LaneInfoSel)1 : Subsystem
  Lane Information Selection (LaneInfoSel)2 : Subsystem
  Saturation1 : Saturate  UpperLimit=0.0117  LowerLimit=0.00237
      settings: AttributesFormatString="Min = %<LowerLimit>  Max = %<UpperLimit>"
  Saturation2 : Saturate  UpperLimit=2  LowerLimit=0.6
      settings: AttributesFormatString="Min = %<LowerLimit>  Max = %<UpperLimit>"
  Saturation3 : Saturate  UpperLimit=150  LowerLimit=60
      settings: AttributesFormatString="Min = %<LowerLimit>  Max = %<UpperLimit>"
  Signal Latching : Subsystem  mask(Signal Latching:){LatchTime=1}
      mask prompts: LatchTime "Latch time(-):"
      mask help:
      | If the latch time is not reached, the input signal will just go through the block. If the latch time is reached, the output will be held and do not change again. The latch time is described with the number of the sampling time.
      | ----vcdc.ascl@jlu 19-01-15
  Signal Latching2 : Subsystem  mask(Signal Latching:){LatchTime=1}
      mask prompts: LatchTime "Latch time(-):"
      mask help:
      | If the latch time is not reached, the input signal will just go through the block. If the latch time is reached, the output will be held and do not change again. The latch time is described with the number of the sampling time.
      | ----vcdc.ascl@jlu 19-01-15
  Signal Latching3 : Subsystem  mask(Signal Latching:){LatchTime=1}
      mask prompts: LatchTime "Latch time(-):"
      mask help:
      | If the latch time is not reached, the input signal will just go through the block. If the latch time is reached, the output will be held and do not change again. The latch time is described with the number of the sampling time.
      | ----vcdc.ascl@jlu 19-01-15
  Signal Latching4 : Subsystem  mask(Signal Latching:){LatchTime=1}
      mask prompts: LatchTime "Latch time(-):"
      mask help:
      | If the latch time is not reached, the input signal will just go through the block. If the latch time is reached, the output will be held and do not change again. The latch time is described with the number of the sampling time.
      | ----vcdc.ascl@jlu 19-01-15
  Signal Latching5 : Subsystem  mask(Signal Latching:){LatchTime=1}
      mask prompts: LatchTime "Latch time(-):"
      mask help:
      | If the latch time is not reached, the input signal will just go through the block. If the latch time is reached, the output will be held and do not change again. The latch time is described with the number of the sampling time.
      | ----vcdc.ascl@jlu 19-01-15
  Signal Latching6 : Subsystem  mask(Signal Latching:){LatchTime=1}
      mask prompts: LatchTime "Latch time(-):"
      mask help:
      | If the latch time is not reached, the input signal will just go through the block. If the latch time is reached, the output will be held and do not change again. The latch time is described with the number of the sampling time.
      | ----vcdc.ascl@jlu 19-01-15
  Signal Latching7 : Subsystem  mask(Signal Latching:){LatchTime=1}
      mask prompts: LatchTime "Latch time(-):"
      mask help:
      | If the latch time is not reached, the input signal will just go through the block. If the latch time is reached, the output will be held and do not change again. The latch time is described with the number of the sampling time.
      | ----vcdc.ascl@jlu 19-01-15
  Subsystem : Subsystem
  MPInP_bsMPInPInfo : Outport
  wires:
  Signal Latching/1(Out) -> Bus Creator/7
  Signal Latching6/1(Out) -> Bus Creator/8  "MPInP_phiSWAIni"
  Bus Selector1/2 -> Lane Information Selection (LaneInfoSel)/3(LaneInfoSel_facmRgtLane)  "<RGTTTLC>"
  Bus Selector1/1 -> Lane Information Selection (LaneInfoSel)/2(LaneInfoSel_facmLftLane)  "<LFTTTLC>"
  Lane Information Selection (LaneInfoSel)/1(LaneInfoSel_facmActvLane) -> Signal Latching5/1(In)
  MPInP_bsLKAInPInfo/1 -> Bus Selector1/1, Bus Selector4/1
  Cast To Single1/1 -> Bus Creator/10  "MPInP_vVehSpd"
  Bus Selector3/1 -> Signal Latching6/1(In)  "<SW_Angle>"
  MPInP_phiHdAgMax/1 -> Signal Latching/1(In)  "MPInP_phiHdAgMax"
  Signal Latching4/1(Out) -> Bus Creator/5  "MPInP_phiHdAgIni"
  Signal Latching2/1(Out) -> Bus Creator/3  "MPInP_phiPrvwHdAgIni"
  Signal Latching3/1(Out) -> Bus Creator/4  "MPInP_lDvtIni"
  MPInP_stLKAActvFlg/1 -> Subsystem/1(In1), Lane Information Selection (LaneInfoSel)2/1(LaneInfoSel_stLKAActvFlg), Lane Information Selection (LaneInfoSel)1/1(LaneInfoSel_stLKAActvFlg), Lane Information Selection (LaneInfoSel)/1(LaneInfoSel_stLKAActvFlg)
  Saturation1/1 -> Bus Creator/11  "StbFacm_SY"
  Signal Latching5/1(Out) -> Saturation2/1  "MPInP_tiTTLCIni"
  Signal Latching7/1(Out) -> Bus Creator/9  "MPInP_vVehSpdIni"
  Bus Selector3/2 -> Signal Latching7/1(In), Saturation3/1, Cast To Single1/1  "<ESC_VehSpd>"
  MPInP_bsInInfoSyn/1 -> Bus Selector3/1
  Subsystem/1(Out6) -> Bus Creator/1  "MPInP_stLDDir"
  Divide1/1 -> Saturation1/1
  Bus Creator/1 -> MPInP_bsMPInPInfo/1
  Saturation2/1 -> Bus Creator/2  "MPInP_tiTTLCIni"
  Constant/1 -> Divide1/1
  Saturation3/1 -> Divide1/2  "Vx"
  Bus Selector4/1 -> Lane Information Selection (LaneInfoSel)1/2(LaneInfoSel_facmLftLane)  "<phiPrvwTTLCHdAgLft>"
  Bus Selector4/2 -> Lane Information Selection (LaneInfoSel)1/3(LaneInfoSel_facmRgtLane)  "<phiPrvwTTLCHdAgRgt>"
  Bus Selector4/3 -> Lane Information Selection (LaneInfoSel)2/2(LaneInfoSel_facmLftLane)  "<lPrvwDvtLft>"
  Bus Selector4/4 -> Lane Information Selection (LaneInfoSel)2/3(LaneInfoSel_facmRgtLane)  "<lPrvwDvtRgt>"
  Bus Selector4/5 -> Signal Latching4/1(In)  "<phiHdAg>"
  Bus Selector4/6 -> Bus Creator/6  "<UndrLim_dphiSWARMax>"
  Lane Information Selection (LaneInfoSel)1/1(LaneInfoSel_facmActvLane) -> Signal Latching2/1(In)
  Lane Information Selection (LaneInfoSel)2/1(LaneInfoSel_facmActvLane) -> Signal Latching3/1(In)

== system LKAS_DFL/LKAS/LL/LLOn/LKA/LKA Motion Planning (LKAMP) /Nominal Time Calculation (NomTCalc) ==
  NomTCalc_vVehSpd : Inport
  NomTCalc_vVehSpdIni : Inport  Port=2
  Add : Sum  OutDataTypeStr=single
  Divide : Product  Inputs=*/  OutDataTypeStr=single
  Gain : Gain  Gain=1/3.6  OutDataTypeStr=single
  Gain1 : Gain  Gain=1/3.6  OutDataTypeStr=single
  Memory : Memory  InheritSampleTime=on
  Product : Product
  NomTCalc_tiNomT : Outport
  wires:
  [LKA_SampleTime] -> Product/2
  Divide/1 -> Add/1
  Product/1 -> Divide/1
  Gain1/1 -> Divide/2
  NomTCalc_vVehSpdIni/1 -> Gain1/1
  Gain/1 -> Product/1
  Memory/1 -> Add/2
  Add/1 -> Memory/1, NomTCalc_tiNomT/1
  NomTCalc_vVehSpd/1 -> Gain/1

== system LKAS_DFL/LKAS/LL/LLOn/LKA/LKA Motion Planning (LKAMP) /Steering Wheel Angle Command Calculation (SWACmdCal) ==
  SWACmdCal_bsK1K2DetOut : Inport
  SWACmdCal_bsLKAInPInfo : Inport  Port=2
  SWACmdCal_tiNomT : Inport  Port=3
  Bus Selector : BusSelector  OutputSignals=K1K2Det_dphi1PhSWAGrad,K1K2Det_phi2PhSWAIni,K1K2Det_dphi2PhSWAGrad1
  Bus Selector1 : BusSelector  OutputSignals=MPInP_phiSWAIni
  SWACmd : MATLAB Function  TreatAsAtomicUnit=on
  SWACmdCal_phiSWACmd : Outport
  SWACmdCal_tiT1 : Outport  Port=2
  SWACmdCal_tiT2 : Outport  Port=3
  wires:
  SWACmd/3(T2) -> SWACmdCal_tiT2/1
  SWACmd/1(SWACmd_phiSWACmd) -> SWACmdCal_phiSWACmd/1
  SWACmdCal_bsK1K2DetOut/1 -> Bus Selector/1
  Bus Selector/2 -> SWACmd/2(SWACmd_phi2PhSWAIni)  "<K1K2Det_phi2PhSWAIni>"
  Bus Selector/3 -> SWACmd/3(SWACmd_dphi2PhSWAGrad)  "<K1K2Det_dphi2PhSWAGrad1>"
  Bus Selector/1 -> SWACmd/1(SWACmd_dphi1PhSWAGrad)  "<K1K2Det_dphi1PhSWAGrad>"
  SWACmdCal_bsLKAInPInfo/1 -> Bus Selector1/1
  Bus Selector1/1 -> SWACmd/4(SWACmd_phi1PhSWAIni)  "<MPInP_phiSWAIni>"
  SWACmdCal_tiNomT/1 -> SWACmd/5(SWACmd_tiNomT)
  SWACmd/2(T1) -> SWACmdCal_tiT1/1

== system LKAS_DFL/LKAS/LL/LLOn/LKA/LKA Motion Planning (LKAMP) /Switching Condition (SwtCon) ==
  SwtCon_stLKAActvFlg : Inport
  SwtCon_bsLKAInPInfo : Inport  Port=2
  SwtCon_vVehSpd : Inport  Port=3
  SwtCon_lLaneWidth_C : Inport  Port=4
  SwtCon_lCarWidth_C : Inport  Port=5
  SwtCon_tiHdAgExTime_C : Inport  Port=6
  SwtCon_tiLSpdCompT_C : Inport  Port=7
  Bus Selector1 : BusSelector  OutputSignals=bsPrCrvtInfo.crPrvwCrvt
  Ending Heading Angle Determination (EndHdAgDet) : Subsystem
  If : If  IfExpression=u1==1  ElseIfExpressions=u1==2
  If Action Subsystem : Subsystem  TreatAsAtomicUnit=on
  If Action Subsystem1 : Subsystem  TreatAsAtomicUnit=on
  If Action Subsystem2 : Subsystem  TreatAsAtomicUnit=on
  Merge : Merge  Inputs=3
  SwtCon_phiHdAgMax : Outport
  wires:
  Bus Selector1/1 -> Ending Heading Angle Determination (EndHdAgDet)/3(EndHdAgDet_crPrvwCrvt)  "<crPrvwCrvt>"
  SwtCon_bsLKAInPInfo/1 -> Bus Selector1/1
  SwtCon_tiLSpdCompT_C/1 -> Ending Heading Angle Determination (EndHdAgDet)/7(EndHdAgDet_tiLSpdCompT_C)
  Merge/1 -> SwtCon_phiHdAgMax/1
  SwtCon_stLKAActvFlg/1 -> Ending Heading Angle Determination (EndHdAgDet)/1(EndHdAgDet_stLKAActvFlg), If/1
  Ending Heading Angle Determination (EndHdAgDet)/1(EndHdAgDet_phiHdAgMax) -> If Action Subsystem/1(In1), If Action Subsystem1/1(In1)
  SwtCon_vVehSpd/1 -> Ending Heading Angle Determination (EndHdAgDet)/2(EndHdAgDet_vVehSpd)
  SwtCon_tiHdAgExTime_C/1 -> Ending Heading Angle Determination (EndHdAgDet)/6(EndHdAgDet_tiHdAgExTime_C)
  SwtCon_lCarWidth_C/1 -> Ending Heading Angle Determination (EndHdAgDet)/5(EndHdAgDet_lCarWidth_C)
  SwtCon_lLaneWidth_C/1 -> Ending Heading Angle Determination (EndHdAgDet)/4(EndHdAgDet_lLaneWidth_C)
  If Action Subsystem2/1(Out1) -> Merge/3
  If/3 -> If Action Subsystem2/Action
  If Action Subsystem1/1(Out1) -> Merge/2
  If/2 -> If Action Subsystem1/Action
  If Action Subsystem/1(Out1) -> Merge/1
  If/1 -> If Action Subsystem/Action

== system LKAS_DFL/LKAS/LL/LLOn/LKA/LKA SWA Limit (LKASWALim)/Rate Limiter Dynamic  ==
  note: Y(k)
  note: U(k)
  up : Inport
  u : Inport  Port=2
  lo : Inport  Port=3
  Add1 : Sum  OutDataTypeStr=uint16
  Constant : Constant  OutDataTypeStr=uint16  SampleTime=-1
  Delay Input2 : UnitDelay  Description=Store in Global RAM  DisableCoverage=on  SampleTime=-1
  Difference Inputs1 : Sum  Description=Add in CPU  DisableCoverage=on  Inputs=+-  OutDataTypeStr=Inherit: Inherit via back propagation
  Difference Inputs2 : Sum  Description=Add in CPU  OutDataTypeStr=Inherit: Inherit via back propagation
  LatchTime_SY : Constant  OutDataTypeStr=uint16  SampleTime=-1
  Memory : Memory  InheritSampleTime=on
  Relational Operator : RelationalOperator  Operator=<=  OutDataTypeStr=boolean  RndMeth=Nearest
  Saturation Dynamic : simulink/Discontinuities/Saturation Dynamic  OutMin=[]  OutMax=[]  OutDataTypeStr=Inherit: Same as second input  OutDataType=fixdt(1, 16)  OutScaling=2^-10  DoSatur=off
  Saturation2 : Saturate  UpperLimit=10000  LowerLimit=0  OutDataTypeStr=uint16
      settings: AttributesFormatString="Min = %<LowerLimit>  Max = %<UpperLimit>"
  Switch : Switch  Criteria=u2 > Threshold
  delta fall limit : Product  DisableCoverage=on  Inputs=**  OutDataTypeStr=Inherit: Inherit via back propagation  SaturateOnIntegerOverflow=on
  delta rise limit : Product  DisableCoverage=on  Inputs=**  OutDataTypeStr=Inherit: Inherit via back propagation  SaturateOnIntegerOverflow=on
  sample time : SampleTimeMath  DisableCoverage=on  TsampMathOp=Ts Only  weightValue=1
  Y : Outport
  wires:
  u/1 -> sample time/1, Switch/1, Difference Inputs1/1
  sample time/1 -> delta fall limit/2, delta rise limit/2
  lo/1 -> delta fall limit/1
  up/1 -> delta rise limit/1
  delta rise limit/1 -> Saturation Dynamic/1
  Difference Inputs2/1 -> Y/1, Delay Input2/1
  Saturation Dynamic/1 -> Difference Inputs2/1
  Switch/1 -> Difference Inputs2/2, Difference Inputs1/2  "Y(k-1)"
  Difference Inputs1/1 -> Saturation Dynamic/2  "( U(k) - Y(k-1) )"
  delta fall limit/1 -> Saturation Dynamic/3
  Add1/1 -> Relational Operator/1, Saturation2/1
  Memory/1 -> Add1/2
  Saturation2/1 -> Memory/1
  LatchTime_SY/1 -> Relational Operator/2
  Constant/1 -> Add1/1
  Relational Operator/1 -> Switch/2
  Delay Input2/1 -> Switch/3  "Y(k-1)"

== system LKAS_DFL/LKAS/LL/LLOn/LKA/Lane Following (LF)/Preview Information Calculation (PIC) ==
  PIC_bsLKAInPInfo : Inport
  Bus Creator1 : BusCreator  Inputs=3
  Bus Selector1 : BusSelector  OutputSignals=bsPrDvtInfo.lPrvwDvtMean,bsPrHdAgInfo.phiPrvwHdAgMean,bsPrCrvtInfo.crPrvwCrvtMean
  PIC_bsPrvwInfo : Outport
  wires:
  Bus Creator1/1 -> PIC_bsPrvwInfo/1
  PIC_bsLKAInPInfo/1 -> Bus Selector1/1
  Bus Selector1/3 -> Bus Creator1/3  "<crPrvwCrvtMean>"
  Bus Selector1/2 -> Bus Creator1/2  "<phiPrvwHdAgMean>"
  Bus Selector1/1 -> Bus Creator1/1  "<lPrvwDvtMean>"

== system LKAS_DFL/LKAS/LL/LLOn/LKA/Lane Following (LF)/Trajectory Following Control (TFC) ==
  TFC_bsPrvwInfo : Inport
  TFC_bsInInfoSyn : Inport  Port=2
  TFC_bsTFCClb : Inport  Port=3
  Bus Selector : BusSelector  OutputSignals=lPrvwDvtMean,phiPrvwHdAgMean,crPrvwCrvtMean
  Bus Selector1 : BusSelector  OutputSignals=bsLKAClb.LL_TFCClb.LL_LFClb_TFC_tiKlatPrvwT_C,bsLKAClb.LL_TFCClb.LL_LFClb_TFC_facmKlat_C,bsLKAClb.LL_TFCClb.LL_LFClb_TFC_vGainLutVehSpdLwr_C,bsLKAClb.LL_TFCClb.LL_LFClb_TFC_vGainLutVehSpdUpr_C,bsLKAClb.LL_TFCClb.LL_LFClb_TFC_facmGainLutGain1_C,bsLKAClb.LL_TFCClb.LL_LFClb_TFC_facmGainLutGain2_C,bsLKAClb.LL_TFCClb.LL_LFClb_TFC_phiIntegCtlMaxSWA_C,bsLKAClb.LL_TFCClb.LL_LFClb_TFC_facmIntegRatio,bsLKAClb.LL_TFCClb.LL_LFClb_TFC_DiffCtrlRatio,bsLKAClb.LL_TFCClb.LL_LFClb_TFC_DiffCtrlMaxSWA,bsLKAClb.LL_TFCClb.LL_LFClb_TFC_DiffCtlBalance,bsLKAClb.LL_TFCClb.LL_LFClb_TFC_FfCtlRatio_C,bsConstantClb.LKA_WhlBaseL_C,bsConstantClb.LKA_StrRatio_C
  Bus Selector3 : BusSelector  OutputSignals=bsLaneInfo.bsL0Info,bsLaneInfo.bsR0Info,bsVehMovInfo.ESC_VehSpd
  Feedback Control (FbCtl) : Subsystem
  Feedforward Control (FfCtl) : Subsystem
  TFC_phiFfSWACmd : Outport
  TFC_phiPropSWACmd : Outport  Port=2
  TFC_phiIntegSWACmd : Outport  Port=3
  TFC_phiDiffSWACmd : Outport  Port=4
  wires:
  Feedback Control (FbCtl)/3(FbCtl_phiFbDiffCtlSWA) -> TFC_phiDiffSWACmd/1
  Bus Selector3/2 -> Feedback Control (FbCtl)/2(FbCtl_bsR0Info)  "<bsR0Info>"
  Bus Selector3/1 -> Feedback Control (FbCtl)/1(FbCtl_bsL0Info)  "<bsL0Info>"
  TFC_bsInInfoSyn/1 -> Bus Selector3/1
  Bus Selector/3 -> Feedforward Control (FfCtl)/3(FfCtl_crPrvwCrvt), Feedback Control (FbCtl)/6(FbCtl_crPrvwCrvt)  "<crPrvwCrvtMean>"
  Feedforward Control (FfCtl)/1(FfCtl_phiFfSWA) -> TFC_phiFfSWACmd/1  "phiFfSWA"
  Feedback Control (FbCtl)/1(FbCtl_phiFbPropCtlSWA) -> TFC_phiPropSWACmd/1
  TFC_bsPrvwInfo/1 -> Bus Selector/1  "bsPrvwInfo"
  Bus Selector/1 -> Feedback Control (FbCtl)/4(FbCtl_lPrvwDvt)  "<lPrvwDvtMean>"
  Bus Selector/2 -> Feedback Control (FbCtl)/5(FbCtl_phiPrvwHdAg)  "<phiPrvwHdAgMean>"
  TFC_bsTFCClb/1 -> Bus Selector1/1
  Bus Selector1/1 -> Feedback Control (FbCtl)/7(FbCtl_tiKlatPrvwT_C)  "<LL_LFClb_TFC_tiKlatPrvwT_C>"
  Bus Selector1/2 -> Feedback Control (FbCtl)/8(FbCtl_facmKlat_C)  "<LL_LFClb_TFC_facmKlat_C>"
  Bus Selector3/3 -> Feedback Control (FbCtl)/3(FbCtl_vVehSpd), Feedforward Control (FfCtl)/2(FfCtl_vVehSpd)  "<ESC_VehSpd>"
  Bus Selector1/3 -> Feedback Control (FbCtl)/9(FbCtl_vVehSpdLimLwr_C)  "<LL_LFClb_TFC_vGainLutVehSpdLwr_C>"
  Bus Selector1/4 -> Feedback Control (FbCtl)/10(FbCtl_vVehSpdLimUpr_C)  "<LL_LFClb_TFC_vGainLutVehSpdUpr_C>"
  Bus Selector1/5 -> Feedback Control (FbCtl)/11(FbCtl_facmGainLimLwr_C)  "<LL_LFClb_TFC_facmGainLutGain1_C>"
  Bus Selector1/6 -> Feedback Control (FbCtl)/12(FbCtl_facmGainLimUpr_C)  "<LL_LFClb_TFC_facmGainLutGain2_C>"
  Bus Selector1/12 -> Feedforward Control (FfCtl)/1(FfCtl_FfCtlRatio_C)  "<LL_LFClb_TFC_FfCtlRatio_C>"
  Bus Selector1/7 -> Feedback Control (FbCtl)/13(FbCtl_phiIntegCtlMaxSWA_C)  "<LL_LFClb_TFC_phiIntegCtlMaxSWA_C>"
  Bus Selector1/8 -> Feedback Control (FbCtl)/14(FbCtl_facmIntegRatio)  "<LL_LFClb_TFC_facmIntegRatio>"
  Feedback Control (FbCtl)/2(FbCtl_phiFbIntegCtlSWA) -> TFC_phiIntegSWACmd/1
  Bus Selector1/10 -> Feedback Control (FbCtl)/16(FbCtl_DiffCtlMaxSWA)  "<LL_LFClb_TFC_DiffCtrlMaxSWA>"
  Bus Selector1/9 -> Feedback Control (FbCtl)/15(FbCtl_DiffCtlRatioIn)  "<LL_LFClb_TFC_DiffCtrlRatio>"
  Bus Selector1/11 -> Feedback Control (FbCtl)/17(FbCtl_DiffCtlBalance)  "<LL_LFClb_TFC_DiffCtlBalance>"
  Bus Selector1/13 -> Feedforward Control (FfCtl)/4(FfCtl_lWhlBase_SY)  "<LKA_WhlBaseL_C>"
  Bus Selector1/14 -> Feedforward Control (FfCtl)/5(FfCtl_rTraRatio_C)  "<LKA_StrRatio_C>"

== system LKAS_DFL/LKAS/LL/LLOn/LKA/Plan To LaneFollowing (PTLF)/InsideJudge ==
  Flg : Inport
  Crvt : Inport  Port=2
  Compare To Constant : simulink/Logic and Bit Operations/Compare To Constant  relop===  const=1  OutDataTypeStr=boolean
  Compare To Constant1 : simulink/Logic and Bit Operations/Compare To Constant  relop===  const=2  OutDataTypeStr=boolean
  Constant : Constant  Value=0.001  OutDataTypeStr=single
  Constant3 : Constant  Value=-0.001  OutDataTypeStr=single
  Logical Operator : Logic  AllPortsSameDT=off  OutDataTypeStr=boolean
  Logical Operator1 : Logic  AllPortsSameDT=off  OutDataTypeStr=boolean
  Logical Operator2 : Logic  Operator=OR  AllPortsSameDT=off  OutDataTypeStr=boolean
  Relational Operator : RelationalOperator  OutDataTypeStr=boolean  RndMeth=Simplest
  Relational Operator1 : RelationalOperator  Operator=<=  OutDataTypeStr=boolean  RndMeth=Simplest
  Out1 : Outport
  wires:
  Compare To Constant/1 -> Logical Operator1/1  "LeftActive"
  Logical Operator1/1 -> Logical Operator2/1
  Logical Operator/1 -> Logical Operator2/2
  Flg/1 -> Compare To Constant1/1, Compare To Constant/1
  Relational Operator/1 -> Logical Operator/2  "RightCrvt"
  Compare To Constant1/1 -> Logical Operator/1  "RightActive"
  Constant/1 -> Relational Operator/2
  Relational Operator1/1 -> Logical Operator1/2  "LeftCrvt"
  Constant3/1 -> Relational Operator1/2
  Logical Operator2/1 -> Out1/1
  Crvt/1 -> Relational Operator1/1, Relational Operator/1

== system LKAS_DFL/LKAS/LL/LLOn/LKA/Plan To LaneFollowing (PTLF)/InsideJudge1 ==
  Flg : Inport
  HdAgLft : Inport  Port=2
  HdAgRgt : Inport  Port=3
  T1 : Inport  Port=4
  Plan : Inport  Port=5
  Time : Inport  Port=6
  If : If  IfExpression=u1 == 1  ElseIfExpressions=u1 == 2
  If Action Subsystem : Subsystem  TreatAsAtomicUnit=on
  If Action Subsystem1 : Subsystem  TreatAsAtomicUnit=on
  If Action Subsystem2 : Subsystem  TreatAsAtomicUnit=on
  Merge : Merge  Inputs=3  InitialOutput=1
  Merge1 : Merge  Inputs=3  InitialOutput=0
  T1_1 : Outport
  Plan_1 : Outport  Port=2
  wires:
  Flg/1 -> If/1
  If/1 -> If Action Subsystem/Action
  If/2 -> If Action Subsystem1/Action
  If/3 -> If Action Subsystem2/Action
  HdAgLft/1 -> If Action Subsystem/3(HdAgLft)
  If Action Subsystem/1(T1_1) -> Merge/1
  If Action Subsystem1/1(T1_1) -> Merge/2
  If Action Subsystem2/1(T1_1) -> Merge/3
  If Action Subsystem/2(Plan_1) -> Merge1/1
  If Action Subsystem1/2(Plan_1) -> Merge1/2
  If Action Subsystem2/2(Plan_1) -> Merge1/3
  T1/1 -> If Action Subsystem/1(T1), If Action Subsystem1/1(T1), If Action Subsystem2/1(T1)
  Plan/1 -> If Action Subsystem/2(Plan), If Action Subsystem1/2(Plan), If Action Subsystem2/2(Plan)
  HdAgRgt/1 -> If Action Subsystem1/3(HdAgRgt)
  Merge/1 -> T1_1/1
  Merge1/1 -> Plan_1/1
  Time/1 -> If Action Subsystem1/4(Time), If Action Subsystem/4(Time)
